simulink model "nid_skeleton_SL"  (Simulink 10.0)
settings: Solver=FixedStepDiscrete  StartTime=0.0  StopTime=inf  RelTol=1e-3  EnableMultiTasking=on
libraries: nid_lib x2
settings Model: Creator=tchikama  LastModifiedBy=bhisma
settings DataIOCC: LimitDataPoints=on  SignalLoggingSaveFormat=ModelDataLogs  SaveOutput=off
settings OptimizationCC: ExpressionDepthLimit=2147483647  SimCompilerOptimization=on
settings DebuggingCC: SolverPrmCheckMsg=warning  FcnCallInpInsideContextMsg=warning  StateNameClashWarn=warning
settings HardwareCC: ProdIntDivRoundTo=Zero  ProdEndianess=LittleEndian  ProdHWDeviceType=Generic->32-bit x86 compatible
settings RTWCC: RTWCompilerOptimization=on
settings CodeAppCC: MaxIdLength=95
settings GRTTargetCC: GeneratePreprocessorConditionals=Disable all
settings ConfigComp: CovExternalEMLEnable=off

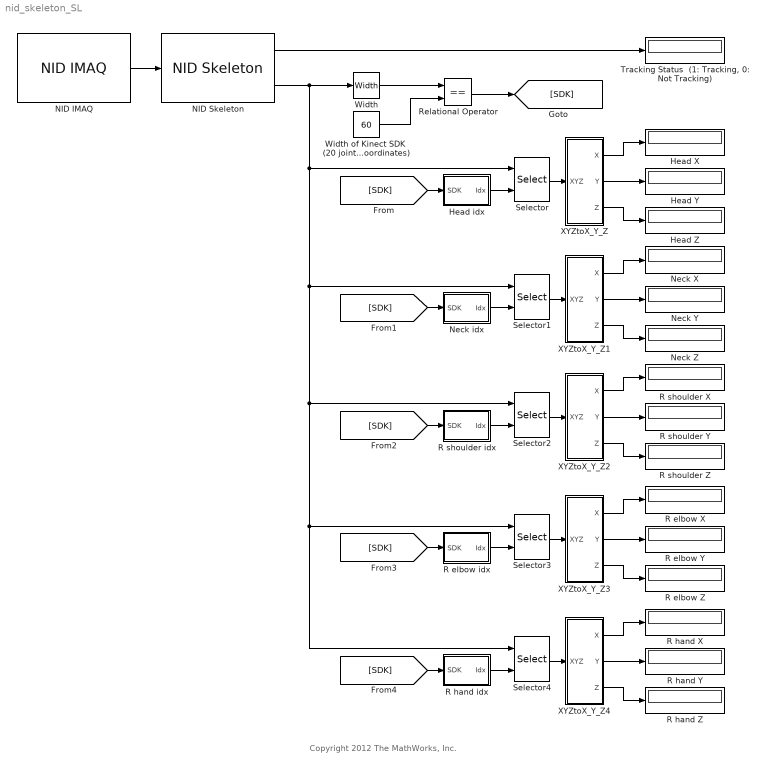
== system nid_skeleton_SL ==
  note: Copyright 2012 The MathWorks, Inc.
  Head X : Display
  Head Y : Display
  Head Z : Display
  Head idx : Subsystem
  NID IMAQ : nid_lib/NID IMAQ  imaq_depth=off  imaq_motion=off  imaq_image=off  view_point=off  imaq_skeleton=on  imaq_ir=off  mirror_image=off  imaq_sample_time=1/30  res_fps=VGA (640x480): 30 FPS  needPsiPose=off  angle=0  angle_read=off  near_mode=off
  NID Skeleton : nid_lib/NID Skeleton  num_of_skeleton_tracking=1  conv_XYZ_RW=on  viewer=off
  Neck X : Display
  Neck Y : Display
  Neck Z : Display
  Neck idx : Subsystem
  R elbow X : Display
  R elbow Y : Display
  R elbow Z : Display
  R elbow idx : Subsystem
  R hand X : Display
  R hand Y : Display
  R hand Z : Display
  R hand idx : Subsystem
  R shoulder X : Display
  R shoulder Y : Display
  R shoulder Z : Display
  R shoulder idx : Subsystem
  Relational Operator : RelationalOperator  Operator===  OutDataTypeStr=boolean  RndMeth=Nearest
  Selector{,1..4} (5 alike) : Selector  NumberOfDimensions=3  InputPortWidth=3  IndexOptions=Select all,Index vector (port),Select all  Indices=[1 3],1,1  OutputSizes=1,1,1
  "Tracking Status  (1: Tracking, 0: Not Tracking)" : Display
  Width : Width
  Width of Kinect SDK  (20 joints x 3 coordinates) : Constant  Value=60
  XYZtoX_Y_Z : Subsystem
  XYZtoX_Y_Z1 : Subsystem
  XYZtoX_Y_Z2 : Subsystem
  XYZtoX_Y_Z3 : Subsystem
  XYZtoX_Y_Z4 : Subsystem
  wires:
  NID IMAQ/1 -> NID Skeleton/1
  Width/1 -> Relational Operator/1
  Width of Kinect SDK  (20 joints x 3 coordinates)/1 -> Relational Operator/2
  NID Skeleton/2 -> Width/1, Selector/1, Selector1/1, Selector2/1, Selector3/1, Selector4/1
  Relational Operator/1 -> [SDK]
  Head idx/1(Idx) -> Selector/2
  [SDK] -> Head idx/1(SDK)
  NID Skeleton/1 -> "Tracking Status  (1: Tracking, 0: Not Tracking)"/1
  Selector/1 -> XYZtoX_Y_Z/1(XYZ)
  XYZtoX_Y_Z/1(X) -> Head X/1
  Neck idx/1(Idx) -> Selector1/2
  [SDK] -> Neck idx/1(SDK)
  Selector1/1 -> XYZtoX_Y_Z1/1(XYZ)
  R shoulder idx/1(Idx) -> Selector2/2
  [SDK] -> R shoulder idx/1(SDK)
  R elbow idx/1(Idx) -> Selector3/2
  [SDK] -> R elbow idx/1(SDK)
  R hand idx/1(Idx) -> Selector4/2
  [SDK] -> R hand idx/1(SDK)
  XYZtoX_Y_Z/2(Y) -> Head Y/1
  XYZtoX_Y_Z/3(Z) -> Head Z/1
  XYZtoX_Y_Z1/1(X) -> Neck X/1
  XYZtoX_Y_Z1/2(Y) -> Neck Y/1
  XYZtoX_Y_Z1/3(Z) -> Neck Z/1
  XYZtoX_Y_Z2/1(X) -> R shoulder X/1
  XYZtoX_Y_Z2/2(Y) -> R shoulder Y/1
  XYZtoX_Y_Z2/3(Z) -> R shoulder Z/1
  Selector2/1 -> XYZtoX_Y_Z2/1(XYZ)
  XYZtoX_Y_Z3/1(X) -> R elbow X/1
  XYZtoX_Y_Z3/2(Y) -> R elbow Y/1
  XYZtoX_Y_Z3/3(Z) -> R elbow Z/1
  Selector3/1 -> XYZtoX_Y_Z3/1(XYZ)
  XYZtoX_Y_Z4/1(X) -> R hand X/1
  XYZtoX_Y_Z4/2(Y) -> R hand Y/1
  XYZtoX_Y_Z4/3(Z) -> R hand Z/1
  Selector4/1 -> XYZtoX_Y_Z4/1(XYZ)

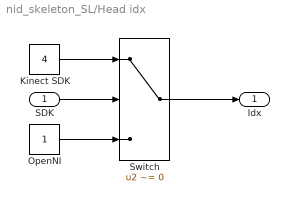
== system nid_skeleton_SL/Head idx ==
  SDK : Inport
  Kinect SDK : Constant  Value=4
  OpenNI : Constant
  Switch : Switch  Criteria=u2 ~= 0
  Idx : Outport
  wires:
  Kinect SDK/1 -> Switch/1
  OpenNI/1 -> Switch/3
  SDK/1 -> Switch/2
  Switch/1 -> Idx/1

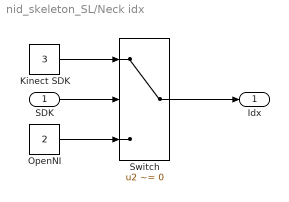
== system nid_skeleton_SL/Neck idx ==
  SDK : Inport
  Kinect SDK : Constant  Value=3
  OpenNI : Constant  Value=2
  Switch : Switch  Criteria=u2 ~= 0
  Idx : Outport
  wires:
  Switch/1 -> Idx/1
  SDK/1 -> Switch/2
  OpenNI/1 -> Switch/3
  Kinect SDK/1 -> Switch/1

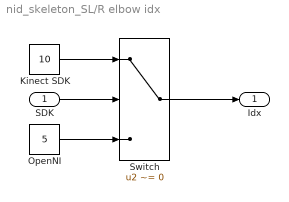
== system nid_skeleton_SL/R elbow idx ==
  SDK : Inport
  Kinect SDK : Constant  Value=10
  OpenNI : Constant  Value=5
  Switch : Switch  Criteria=u2 ~= 0
  Idx : Outport
  wires:
  Kinect SDK/1 -> Switch/1
  OpenNI/1 -> Switch/3
  SDK/1 -> Switch/2
  Switch/1 -> Idx/1

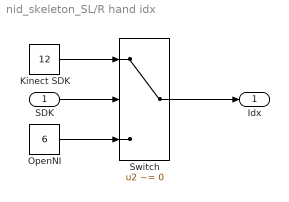
== system nid_skeleton_SL/R hand idx ==
  SDK : Inport
  Kinect SDK : Constant  Value=12
  OpenNI : Constant  Value=6
  Switch : Switch  Criteria=u2 ~= 0
  Idx : Outport
  wires:
  Kinect SDK/1 -> Switch/1
  OpenNI/1 -> Switch/3
  SDK/1 -> Switch/2
  Switch/1 -> Idx/1

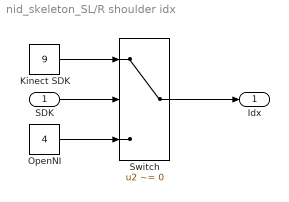
== system nid_skeleton_SL/R shoulder idx ==
  SDK : Inport
  Kinect SDK : Constant  Value=9
  OpenNI : Constant  Value=4
  Switch : Switch  Criteria=u2 ~= 0
  Idx : Outport
  wires:
  Kinect SDK/1 -> Switch/1
  OpenNI/1 -> Switch/3
  SDK/1 -> Switch/2
  Switch/1 -> Idx/1

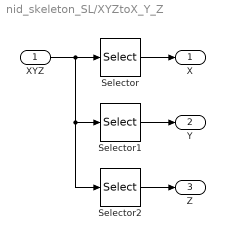
== system nid_skeleton_SL/XYZtoX_Y_Z ==
  XYZ : Inport
  Selector : Selector  NumberOfDimensions=3  InputPortWidth=3  IndexOptions=Index vector (dialog),Index vector (dialog),Index vector (dialog)  Indices=1,1,1  OutputSizes=1,1,1
  Selector1 : Selector  NumberOfDimensions=3  InputPortWidth=3  IndexOptions=Index vector (dialog),Index vector (dialog),Index vector (dialog)  Indices=1,1,2  OutputSizes=1,1,1
  Selector2 : Selector  NumberOfDimensions=3  InputPortWidth=3  IndexOptions=Index vector (dialog),Index vector (dialog),Index vector (dialog)  Indices=1,1,3  OutputSizes=1,1,1
  X : Outport
  Y : Outport  Port=2
  Z : Outport  Port=3
  wires:
  XYZ/1 -> Selector/1, Selector1/1, Selector2/1
  Selector/1 -> X/1
  Selector1/1 -> Y/1
  Selector2/1 -> Z/1

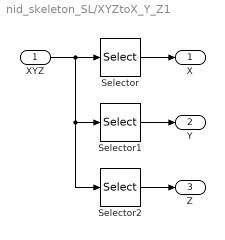
== system nid_skeleton_SL/XYZtoX_Y_Z1 ==
  XYZ : Inport
  Selector : Selector  NumberOfDimensions=3  InputPortWidth=3  IndexOptions=Index vector (dialog),Index vector (dialog),Index vector (dialog)  Indices=1,1,1  OutputSizes=1,1,1
  Selector1 : Selector  NumberOfDimensions=3  InputPortWidth=3  IndexOptions=Index vector (dialog),Index vector (dialog),Index vector (dialog)  Indices=1,1,2  OutputSizes=1,1,1
  Selector2 : Selector  NumberOfDimensions=3  InputPortWidth=3  IndexOptions=Index vector (dialog),Index vector (dialog),Index vector (dialog)  Indices=1,1,3  OutputSizes=1,1,1
  X : Outport
  Y : Outport  Port=2
  Z : Outport  Port=3
  wires:
  Selector2/1 -> Z/1
  Selector1/1 -> Y/1
  Selector/1 -> X/1
  XYZ/1 -> Selector2/1, Selector1/1, Selector/1

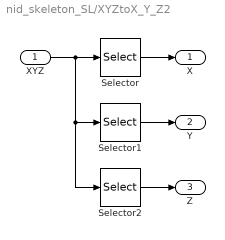
== system nid_skeleton_SL/XYZtoX_Y_Z2 ==
  XYZ : Inport
  Selector : Selector  NumberOfDimensions=3  InputPortWidth=3  IndexOptions=Index vector (dialog),Index vector (dialog),Index vector (dialog)  Indices=1,1,1  OutputSizes=1,1,1
  Selector1 : Selector  NumberOfDimensions=3  InputPortWidth=3  IndexOptions=Index vector (dialog),Index vector (dialog),Index vector (dialog)  Indices=1,1,2  OutputSizes=1,1,1
  Selector2 : Selector  NumberOfDimensions=3  InputPortWidth=3  IndexOptions=Index vector (dialog),Index vector (dialog),Index vector (dialog)  Indices=1,1,3  OutputSizes=1,1,1
  X : Outport
  Y : Outport  Port=2
  Z : Outport  Port=3
  wires:
  XYZ/1 -> Selector/1, Selector1/1, Selector2/1
  Selector/1 -> X/1
  Selector1/1 -> Y/1
  Selector2/1 -> Z/1

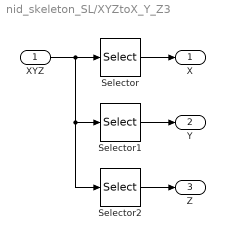
== system nid_skeleton_SL/XYZtoX_Y_Z3 ==
  XYZ : Inport
  Selector : Selector  NumberOfDimensions=3  InputPortWidth=3  IndexOptions=Index vector (dialog),Index vector (dialog),Index vector (dialog)  Indices=1,1,1  OutputSizes=1,1,1
  Selector1 : Selector  NumberOfDimensions=3  InputPortWidth=3  IndexOptions=Index vector (dialog),Index vector (dialog),Index vector (dialog)  Indices=1,1,2  OutputSizes=1,1,1
  Selector2 : Selector  NumberOfDimensions=3  InputPortWidth=3  IndexOptions=Index vector (dialog),Index vector (dialog),Index vector (dialog)  Indices=1,1,3  OutputSizes=1,1,1
  X : Outport
  Y : Outport  Port=2
  Z : Outport  Port=3
  wires:
  Selector2/1 -> Z/1
  Selector1/1 -> Y/1
  Selector/1 -> X/1
  XYZ/1 -> Selector2/1, Selector1/1, Selector/1

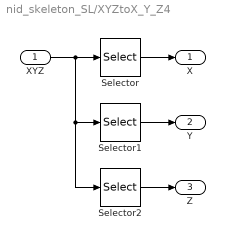
== system nid_skeleton_SL/XYZtoX_Y_Z4 ==
  XYZ : Inport
  Selector : Selector  NumberOfDimensions=3  InputPortWidth=3  IndexOptions=Index vector (dialog),Index vector (dialog),Index vector (dialog)  Indices=1,1,1  OutputSizes=1,1,1
  Selector1 : Selector  NumberOfDimensions=3  InputPortWidth=3  IndexOptions=Index vector (dialog),Index vector (dialog),Index vector (dialog)  Indices=1,1,2  OutputSizes=1,1,1
  Selector2 : Selector  NumberOfDimensions=3  InputPortWidth=3  IndexOptions=Index vector (dialog),Index vector (dialog),Index vector (dialog)  Indices=1,1,3  OutputSizes=1,1,1
  X : Outport
  Y : Outport  Port=2
  Z : Outport  Port=3
  wires:
  XYZ/1 -> Selector/1, Selector1/1, Selector2/1
  Selector/1 -> X/1
  Selector1/1 -> Y/1
  Selector2/1 -> Z/1
